simulink model "untitled1"  (R2024b)
settings: Solver=VariableStepAuto  StartTime=0.0  StopTime=10.0  RelTol=1e-3
undefined symbols (not defined in the file): control, controlParams, ControlSampleTime, CriticalTiltAngle, DiscIntNeverNeededParam, dspblkCoreblockFVToolHelper, flightState, FWControlParams, FWTrimSpeed, gcbh, ReferenceFilterDen, ReferenceFilterNum, tilt_max, tilt_trim, TiltScheduleRate, uavParam, w_trim, WindDownRate
libraries: slpidlib x31, simulink x9
(part 2 of 5)

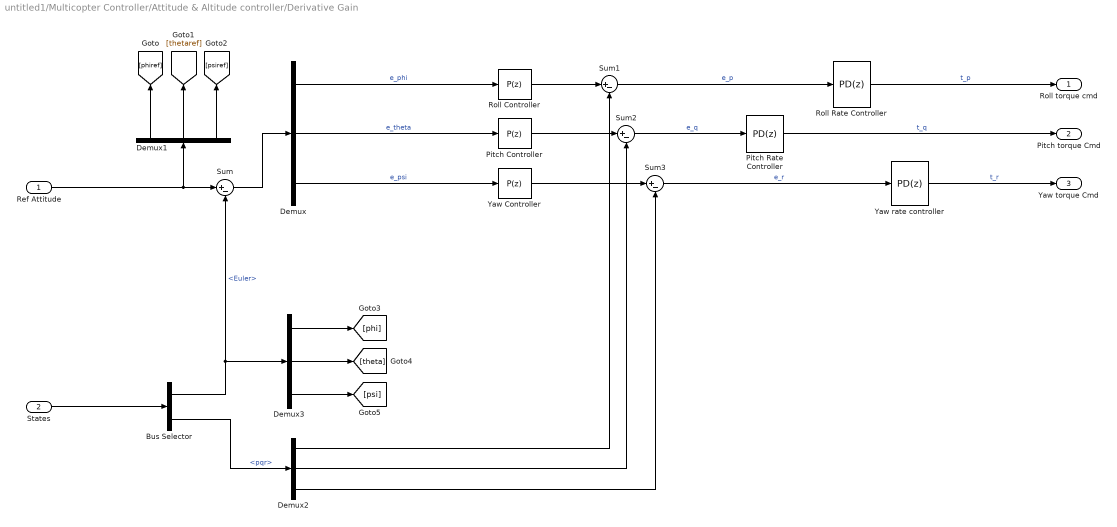
== system untitled1/Multicopter Controller/Attitude & Altitude controller/Derivative Gain ==
  Ref Attitude : Inport
  States : Inport  Port=2
  Bus Selector : BusSelector  OutputSignals=Euler,pqr
  Demux{,1..3} (4 alike) : Demux  Outputs=3
  Pitch Controller : slpidlib/PID Controller  Controller=P  Form=Parallel  TimeDomain=Discrete-time  UseExternalTs=off  SampleTime=0.005  IntegratorMethod=Forward Euler  FilterMethod=Forward Euler  ControllerParametersSource=internal  P=controlParams.P_PITCH  I=0.005  UseKiTs=on  D=1.47243904216696  UseExternalDerivativeSource=off  N=36.4796619058829  UseFilter=on  TunerSelectOption=Transfer Function Based (PID Tuner App)  InitialConditionSource=internal  InitialConditionForIntegrator=0  InitialConditionForFilter=0  DifferentiatorICPrevScaledInput=0  ExternalReset=none  TrackingMode=off  Kt=1  LimitOutput=off  SatLimitsSource=internal  UpperSaturationLimit=inf  LowerSaturationLimit=-inf  LinearizeAsGain=on  AntiWindupMode=none  Kb=1  LimitIntegrator=off  UpperIntegratorSaturationLimit=inf  LowerIntegratorSaturationLimit=-inf  POutMin=[]  POutMax=[]  IOutMin=[]  IOutMax=[]  DOutMin=[]  DOutMax=[]  NOutMin=[]  NOutMax=[]  SumOutMin=[]  SumOutMax=[]  SaturationOutMin=[]  SaturationOutMax=[]  PParamMin=[]  PParamMax=[]  IParamMin=[]  IParamMax=[]  DParamMin=[]  DParamMax=[]  NParamMin=[]  NParamMax=[]  KbParamMin=[]  KbParamMax=[]  KtParamMin=[]  KtParamMax=[]  KbOutMin=[]  KbOutMax=[]  KtOutMin=[]  KtOutMax=[]  IntegratorOutMin=[]  IntegratorOutMax=[]  FilterOutMin=[]  FilterOutMax=[]  SumI1OutMin=[]  SumI1OutMax=[]  SumI2OutMin=[]  SumI2OutMax=[]  SumI3OutMin=[]  SumI3OutMax=[]  SumI4OutMin=[]  SumI4OutMax=[]  SumDOutMin=[]  SumDOutMax=[]  DifferentiatorOutMin=[]  DifferentiatorOutMax=[]  FilterDiffOutCoefMin=[]  FilterDiffOutCoefMax=[]  ReciprocalOutMin=[]  ReciprocalOutMax=[]  SumDenOutMin=[]  SumDenOutMax=[]  SumNumOutMin=[]  SumNumOutMax=[]  DivideOutMin=[]  DivideOutMax=[]  UdiffTsProdOutMin=[]  UdiffTsProdOutMax=[]  NTsProdOutMin=[]  NTsProdOutMax=[]  UintegralTsProdOutMin=[]  UintegralTsProdOutMax=[]  UngainTsProdOutMin=[]  UngainTsProdOutMax=[]  ClampingZeroOutDataTypeStr=Inherit: Inherit via back propagation  ClampingZeroOutMin=[]  ClampingZeroOutMax=[]  FilterDenConstantOutDataTypeStr=Inherit: Inherit via back propagation  FilterDenConstantOutMin=[]  FilterDenConstantOutMax=[]  PCopyOutDataTypeStr=Inherit: Inherit via back propagation  PCopyOutMin=[]  PCopyOutMax=[]  NCopyOutDataTypeStr=Inherit: Inherit via back propagation  NCopyOutMin=[]  NCopyOutMax=[]  IntegratorContinuousStateAttributes=''  IntegratorStateMustResolveToSignalObject=off  IntegratorRTWStateStorageClass=Auto  FilterContinuousStateAttributes=''  FilterStateMustResolveToSignalObject=off  FilterRTWStateStorageClass=Auto  ParallelPVariant=InternalParameters  IdealPVariant=Disabled  IVariant=Disabled  DVariant=Disabled  IntegratorVariant=Disabled  SatVariant=Disabled  AWVariant=Disabled  PCopyVariant=Disabled  TRVariant=Disabled  FdbkBlocksVariant=Forward  IdealPFdbkVariant=Disabled  SatFdbkVariant=Disabled  DerivativeFilterVariant=Disabled  NVariant=Disabled  NCopyVariant=Disabled_SignalSpec  FilterICVariant=Disabled  IntegratorICVariant=Disabled  ExternalResetVariant=Disabled  TRSumVariant=Passthrough  SumFdbkVariant=Disabled  SumVariant=Passthrough_P  TsampFilterVariant=InternalTs  TsampNgainVariant=Passthrough  TsampIntegralVariant=Disabled_SignalSpec  ExternalSaturationOutDataTypeStr=Inherit: Same as second input  DerivativeSourceVariant=Disabled  PreIntVariant=InternalPreInt
  Pitch Rate Controller : slpidlib/PID Controller  Controller=PD  Form=Parallel  TimeDomain=Discrete-time  UseExternalTs=off  SampleTime=0.005  IntegratorMethod=Forward Euler  FilterMethod=Forward Euler  ControllerParametersSource=internal  P=controlParams.P_PITCH_RATE  I=controlParams.I_PITCH_RATE*0  UseKiTs=off  D=controlParams.D_PITCH_RATE  UseExternalDerivativeSource=off  N=controlParams.N_PITCH_RATE  UseFilter=on  TunerSelectOption=Transfer Function Based (PID Tuner App)  InitialConditionSource=internal  InitialConditionForIntegrator=0  InitialConditionForFilter=0  DifferentiatorICPrevScaledInput=0  ExternalReset=none  TrackingMode=off  Kt=1  LimitOutput=off  SatLimitsSource=internal  UpperSaturationLimit=inf  LowerSaturationLimit=-inf  LinearizeAsGain=on  AntiWindupMode=none  Kb=1  LimitIntegrator=off  UpperIntegratorSaturationLimit=inf  LowerIntegratorSaturationLimit=-inf  POutMin=[]  POutMax=[]  IOutMin=[]  IOutMax=[]  DOutMin=[]  DOutMax=[]  NOutMin=[]  NOutMax=[]  SumOutMin=[]  SumOutMax=[]  SaturationOutMin=[]  SaturationOutMax=[]  PParamMin=[]  PParamMax=[]  IParamMin=[]  IParamMax=[]  DParamMin=[]  DParamMax=[]  NParamMin=[]  NParamMax=[]  KbParamMin=[]  KbParamMax=[]  KtParamMin=[]  KtParamMax=[]  KbOutMin=[]  KbOutMax=[]  KtOutMin=[]  KtOutMax=[]  IntegratorOutMin=[]  IntegratorOutMax=[]  FilterOutMin=[]  FilterOutMax=[]  SumI1OutMin=[]  SumI1OutMax=[]  SumI2OutMin=[]  SumI2OutMax=[]  SumI3OutMin=[]  SumI3OutMax=[]  SumI4OutMin=[]  SumI4OutMax=[]  SumDOutMin=[]  SumDOutMax=[]  DifferentiatorOutMin=[]  DifferentiatorOutMax=[]  FilterDiffOutCoefMin=[]  FilterDiffOutCoefMax=[]  ReciprocalOutMin=[]  ReciprocalOutMax=[]  SumDenOutMin=[]  SumDenOutMax=[]  SumNumOutMin=[]  SumNumOutMax=[]  DivideOutMin=[]  DivideOutMax=[]  UdiffTsProdOutMin=[]  UdiffTsProdOutMax=[]  NTsProdOutMin=[]  NTsProdOutMax=[]  UintegralTsProdOutMin=[]  UintegralTsProdOutMax=[]  UngainTsProdOutMin=[]  UngainTsProdOutMax=[]  ClampingZeroOutDataTypeStr=Inherit: Inherit via back propagation  ClampingZeroOutMin=[]  ClampingZeroOutMax=[]  FilterDenConstantOutDataTypeStr=Inherit: Inherit via back propagation  FilterDenConstantOutMin=[]  FilterDenConstantOutMax=[]  PCopyOutDataTypeStr=Inherit: Inherit via back propagation  PCopyOutMin=[]  PCopyOutMax=[]  NCopyOutDataTypeStr=Inherit: Inherit via back propagation  NCopyOutMin=[]  NCopyOutMax=[]  IntegratorContinuousStateAttributes=''  IntegratorStateMustResolveToSignalObject=off  IntegratorRTWStateStorageClass=Auto  FilterContinuousStateAttributes=''  FilterStateMustResolveToSignalObject=off  FilterRTWStateStorageClass=Auto  ParallelPVariant=InternalParameters  IdealPVariant=Disabled  IVariant=Disabled  DVariant=InternalParameters  IntegratorVariant=Disabled  SatVariant=Disabled  AWVariant=Disabled  PCopyVariant=Disabled  TRVariant=Disabled  FdbkBlocksVariant=Forward  IdealPFdbkVariant=Disabled  SatFdbkVariant=Disabled  DerivativeFilterVariant=ForwardEulerFilter  NVariant=InternalParameters  NCopyVariant=Disabled  FilterICVariant=InternalICsFilter  IntegratorICVariant=Disabled  ExternalResetVariant=Disabled  TRSumVariant=Passthrough  SumFdbkVariant=Disabled  SumVariant=Sum_PD  TsampFilterVariant=InternalTs  TsampNgainVariant=Passthrough  TsampIntegralVariant=Disabled_SignalSpec  ExternalSaturationOutDataTypeStr=Inherit: Same as second input  DerivativeSourceVariant=ErrorSignal  PreIntVariant=InternalPreInt
  Roll Controller : slpidlib/PID Controller  Controller=P  Form=Parallel  TimeDomain=Discrete-time  UseExternalTs=off  SampleTime=0.005  IntegratorMethod=Forward Euler  FilterMethod=Forward Euler  ControllerParametersSource=internal  P=controlParams.P_ROLL  I=0.005  UseKiTs=on  D=0.952146167984845  UseExternalDerivativeSource=off  N=4.97655809990509  UseFilter=on  TunerSelectOption=Transfer Function Based (PID Tuner App)  InitialConditionSource=internal  InitialConditionForIntegrator=0  InitialConditionForFilter=0  DifferentiatorICPrevScaledInput=0  ExternalReset=none  TrackingMode=off  Kt=1  LimitOutput=off  SatLimitsSource=internal  UpperSaturationLimit=inf  LowerSaturationLimit=-inf  LinearizeAsGain=on  AntiWindupMode=none  Kb=1  LimitIntegrator=off  UpperIntegratorSaturationLimit=inf  LowerIntegratorSaturationLimit=-inf  POutMin=[]  POutMax=[]  IOutMin=[]  IOutMax=[]  DOutMin=[]  DOutMax=[]  NOutMin=[]  NOutMax=[]  SumOutMin=[]  SumOutMax=[]  SaturationOutMin=[]  SaturationOutMax=[]  PParamMin=[]  PParamMax=[]  IParamMin=[]  IParamMax=[]  DParamMin=[]  DParamMax=[]  NParamMin=[]  NParamMax=[]  KbParamMin=[]  KbParamMax=[]  KtParamMin=[]  KtParamMax=[]  KbOutMin=[]  KbOutMax=[]  KtOutMin=[]  KtOutMax=[]  IntegratorOutMin=[]  IntegratorOutMax=[]  FilterOutMin=[]  FilterOutMax=[]  SumI1OutMin=[]  SumI1OutMax=[]  SumI2OutMin=[]  SumI2OutMax=[]  SumI3OutMin=[]  SumI3OutMax=[]  SumI4OutMin=[]  SumI4OutMax=[]  SumDOutMin=[]  SumDOutMax=[]  DifferentiatorOutMin=[]  DifferentiatorOutMax=[]  FilterDiffOutCoefMin=[]  FilterDiffOutCoefMax=[]  ReciprocalOutMin=[]  ReciprocalOutMax=[]  SumDenOutMin=[]  SumDenOutMax=[]  SumNumOutMin=[]  SumNumOutMax=[]  DivideOutMin=[]  DivideOutMax=[]  UdiffTsProdOutMin=[]  UdiffTsProdOutMax=[]  NTsProdOutMin=[]  NTsProdOutMax=[]  UintegralTsProdOutMin=[]  UintegralTsProdOutMax=[]  UngainTsProdOutMin=[]  UngainTsProdOutMax=[]  ClampingZeroOutDataTypeStr=Inherit: Inherit via back propagation  ClampingZeroOutMin=[]  ClampingZeroOutMax=[]  FilterDenConstantOutDataTypeStr=Inherit: Inherit via back propagation  FilterDenConstantOutMin=[]  FilterDenConstantOutMax=[]  PCopyOutDataTypeStr=Inherit: Inherit via back propagation  PCopyOutMin=[]  PCopyOutMax=[]  NCopyOutDataTypeStr=Inherit: Inherit via back propagation  NCopyOutMin=[]  NCopyOutMax=[]  IntegratorContinuousStateAttributes=''  IntegratorStateMustResolveToSignalObject=off  IntegratorRTWStateStorageClass=Auto  FilterContinuousStateAttributes=''  FilterStateMustResolveToSignalObject=off  FilterRTWStateStorageClass=Auto  ParallelPVariant=InternalParameters  IdealPVariant=Disabled  IVariant=Disabled  DVariant=Disabled  IntegratorVariant=Disabled  SatVariant=Disabled  AWVariant=Disabled  PCopyVariant=Disabled  TRVariant=Disabled  FdbkBlocksVariant=Forward  IdealPFdbkVariant=Disabled  SatFdbkVariant=Disabled  DerivativeFilterVariant=Disabled  NVariant=Disabled  NCopyVariant=Disabled_SignalSpec  FilterICVariant=Disabled  IntegratorICVariant=Disabled  ExternalResetVariant=Disabled  TRSumVariant=Passthrough  SumFdbkVariant=Disabled  SumVariant=Passthrough_P  TsampFilterVariant=InternalTs  TsampNgainVariant=Passthrough  TsampIntegralVariant=Disabled_SignalSpec  ExternalSaturationOutDataTypeStr=Inherit: Same as second input  DerivativeSourceVariant=Disabled  PreIntVariant=InternalPreInt
  Roll Rate Controller : slpidlib/PID Controller  Controller=PD  Form=Parallel  TimeDomain=Discrete-time  UseExternalTs=off  SampleTime=-1  IntegratorMethod=Forward Euler  FilterMethod=Forward Euler  ControllerParametersSource=internal  P=controlParams.P_ROLL_RATE  I=controlParams.I_ROLL_RATE  UseKiTs=off  D=controlParams.D_ROLL_RATE  UseExternalDerivativeSource=off  N=controlParams.N_ROLL_RATE  UseFilter=on  TunerSelectOption=Transfer Function Based (PID Tuner App)  InitialConditionSource=internal  InitialConditionForIntegrator=0  InitialConditionForFilter=0  DifferentiatorICPrevScaledInput=0  ExternalReset=none  TrackingMode=off  Kt=1  LimitOutput=off  SatLimitsSource=internal  UpperSaturationLimit=inf  LowerSaturationLimit=-inf  LinearizeAsGain=on  AntiWindupMode=none  Kb=1  LimitIntegrator=off  UpperIntegratorSaturationLimit=inf  LowerIntegratorSaturationLimit=-inf  POutMin=[]  POutMax=[]  IOutMin=[]  IOutMax=[]  DOutMin=[]  DOutMax=[]  NOutMin=[]  NOutMax=[]  SumOutMin=[]  SumOutMax=[]  SaturationOutMin=[]  SaturationOutMax=[]  PParamMin=[]  PParamMax=[]  IParamMin=[]  IParamMax=[]  DParamMin=[]  DParamMax=[]  NParamMin=[]  NParamMax=[]  KbParamMin=[]  KbParamMax=[]  KtParamMin=[]  KtParamMax=[]  KbOutMin=[]  KbOutMax=[]  KtOutMin=[]  KtOutMax=[]  IntegratorOutMin=[]  IntegratorOutMax=[]  FilterOutMin=[]  FilterOutMax=[]  SumI1OutMin=[]  SumI1OutMax=[]  SumI2OutMin=[]  SumI2OutMax=[]  SumI3OutMin=[]  SumI3OutMax=[]  SumI4OutMin=[]  SumI4OutMax=[]  SumDOutMin=[]  SumDOutMax=[]  DifferentiatorOutMin=[]  DifferentiatorOutMax=[]  FilterDiffOutCoefMin=[]  FilterDiffOutCoefMax=[]  ReciprocalOutMin=[]  ReciprocalOutMax=[]  SumDenOutMin=[]  SumDenOutMax=[]  SumNumOutMin=[]  SumNumOutMax=[]  DivideOutMin=[]  DivideOutMax=[]  UdiffTsProdOutMin=[]  UdiffTsProdOutMax=[]  NTsProdOutMin=[]  NTsProdOutMax=[]  UintegralTsProdOutMin=[]  UintegralTsProdOutMax=[]  UngainTsProdOutMin=[]  UngainTsProdOutMax=[]  ClampingZeroOutDataTypeStr=Inherit: Inherit via back propagation  ClampingZeroOutMin=[]  ClampingZeroOutMax=[]  FilterDenConstantOutDataTypeStr=Inherit: Inherit via back propagation  FilterDenConstantOutMin=[]  FilterDenConstantOutMax=[]  PCopyOutDataTypeStr=Inherit: Inherit via back propagation  PCopyOutMin=[]  PCopyOutMax=[]  NCopyOutDataTypeStr=Inherit: Inherit via back propagation  NCopyOutMin=[]  NCopyOutMax=[]  IntegratorContinuousStateAttributes=''  IntegratorStateMustResolveToSignalObject=off  IntegratorRTWStateStorageClass=Auto  FilterContinuousStateAttributes=''  FilterStateMustResolveToSignalObject=off  FilterRTWStateStorageClass=Auto  ParallelPVariant=InternalParameters  IdealPVariant=Disabled  IVariant=Disabled  DVariant=InternalParameters  IntegratorVariant=Disabled  SatVariant=Disabled  AWVariant=Disabled  PCopyVariant=Disabled  TRVariant=Disabled  FdbkBlocksVariant=Forward  IdealPFdbkVariant=Disabled  SatFdbkVariant=Disabled  DerivativeFilterVariant=ForwardEulerFilter  NVariant=InternalParameters  NCopyVariant=Disabled  FilterICVariant=InternalICsFilter  IntegratorICVariant=Disabled  ExternalResetVariant=Disabled  TRSumVariant=Passthrough  SumFdbkVariant=Disabled  SumVariant=Sum_PD  TsampFilterVariant=InternalTs  TsampNgainVariant=Passthrough  TsampIntegralVariant=Disabled_SignalSpec  ExternalSaturationOutDataTypeStr=Inherit: Same as second input  DerivativeSourceVariant=ErrorSignal  PreIntVariant=InternalPreInt
  Sum{,1..3} (4 alike) : Sum  Inputs=|+-
  Yaw Controller : slpidlib/PID Controller  Controller=P  Form=Parallel  TimeDomain=Discrete-time  UseExternalTs=off  SampleTime=-1  IntegratorMethod=Forward Euler  FilterMethod=Forward Euler  ControllerParametersSource=internal  P=controlParams.P_YAW  I=0.005  UseKiTs=off  D=1.48888612768425  UseExternalDerivativeSource=off  N=213.334111142952  UseFilter=on  TunerSelectOption=Transfer Function Based (PID Tuner App)  InitialConditionSource=internal  InitialConditionForIntegrator=0  InitialConditionForFilter=0  DifferentiatorICPrevScaledInput=0  ExternalReset=none  TrackingMode=off  Kt=1  LimitOutput=off  SatLimitsSource=internal  UpperSaturationLimit=inf  LowerSaturationLimit=-inf  LinearizeAsGain=on  AntiWindupMode=none  Kb=1  LimitIntegrator=off  UpperIntegratorSaturationLimit=inf  LowerIntegratorSaturationLimit=-inf  POutMin=[]  POutMax=[]  IOutMin=[]  IOutMax=[]  DOutMin=[]  DOutMax=[]  NOutMin=[]  NOutMax=[]  SumOutMin=[]  SumOutMax=[]  SaturationOutMin=[]  SaturationOutMax=[]  PParamMin=[]  PParamMax=[]  IParamMin=[]  IParamMax=[]  DParamMin=[]  DParamMax=[]  NParamMin=[]  NParamMax=[]  KbParamMin=[]  KbParamMax=[]  KtParamMin=[]  KtParamMax=[]  KbOutMin=[]  KbOutMax=[]  KtOutMin=[]  KtOutMax=[]  IntegratorOutMin=[]  IntegratorOutMax=[]  FilterOutMin=[]  FilterOutMax=[]  SumI1OutMin=[]  SumI1OutMax=[]  SumI2OutMin=[]  SumI2OutMax=[]  SumI3OutMin=[]  SumI3OutMax=[]  SumI4OutMin=[]  SumI4OutMax=[]  SumDOutMin=[]  SumDOutMax=[]  DifferentiatorOutMin=[]  DifferentiatorOutMax=[]  FilterDiffOutCoefMin=[]  FilterDiffOutCoefMax=[]  ReciprocalOutMin=[]  ReciprocalOutMax=[]  SumDenOutMin=[]  SumDenOutMax=[]  SumNumOutMin=[]  SumNumOutMax=[]  DivideOutMin=[]  DivideOutMax=[]  UdiffTsProdOutMin=[]  UdiffTsProdOutMax=[]  NTsProdOutMin=[]  NTsProdOutMax=[]  UintegralTsProdOutMin=[]  UintegralTsProdOutMax=[]  UngainTsProdOutMin=[]  UngainTsProdOutMax=[]  ClampingZeroOutDataTypeStr=Inherit: Inherit via back propagation  ClampingZeroOutMin=[]  ClampingZeroOutMax=[]  FilterDenConstantOutDataTypeStr=Inherit: Inherit via back propagation  FilterDenConstantOutMin=[]  FilterDenConstantOutMax=[]  PCopyOutDataTypeStr=Inherit: Inherit via back propagation  PCopyOutMin=[]  PCopyOutMax=[]  NCopyOutDataTypeStr=Inherit: Inherit via back propagation  NCopyOutMin=[]  NCopyOutMax=[]  IntegratorContinuousStateAttributes=''  IntegratorStateMustResolveToSignalObject=off  IntegratorRTWStateStorageClass=Auto  FilterContinuousStateAttributes=''  FilterStateMustResolveToSignalObject=off  FilterRTWStateStorageClass=Auto  ParallelPVariant=InternalParameters  IdealPVariant=Disabled  IVariant=Disabled  DVariant=Disabled  IntegratorVariant=Disabled  SatVariant=Disabled  AWVariant=Disabled  PCopyVariant=Disabled  TRVariant=Disabled  FdbkBlocksVariant=Forward  IdealPFdbkVariant=Disabled  SatFdbkVariant=Disabled  DerivativeFilterVariant=Disabled  NVariant=Disabled  NCopyVariant=Disabled_SignalSpec  FilterICVariant=Disabled  IntegratorICVariant=Disabled  ExternalResetVariant=Disabled  TRSumVariant=Passthrough  SumFdbkVariant=Disabled  SumVariant=Passthrough_P  TsampFilterVariant=InternalTs  TsampNgainVariant=Passthrough  TsampIntegralVariant=Disabled_SignalSpec  ExternalSaturationOutDataTypeStr=Inherit: Same as second input  DerivativeSourceVariant=Disabled  PreIntVariant=InternalPreInt
  Yaw rate controller : slpidlib/PID Controller  Controller=PD  Form=Parallel  TimeDomain=Discrete-time  UseExternalTs=off  SampleTime=-1  IntegratorMethod=Forward Euler  FilterMethod=Forward Euler  ControllerParametersSource=internal  P=controlParams.P_YAW_RATE  I=controlParams.I_YAW_RATE  UseKiTs=off  D=controlParams.D_YAW_RATE  UseExternalDerivativeSource=off  N=controlParams.N_YAW_RATE  UseFilter=on  TunerSelectOption=Transfer Function Based (PID Tuner App)  InitialConditionSource=internal  InitialConditionForIntegrator=0  InitialConditionForFilter=0  DifferentiatorICPrevScaledInput=0  ExternalReset=none  TrackingMode=off  Kt=1  LimitOutput=off  SatLimitsSource=internal  UpperSaturationLimit=inf  LowerSaturationLimit=-inf  LinearizeAsGain=on  AntiWindupMode=none  Kb=1  LimitIntegrator=off  UpperIntegratorSaturationLimit=inf  LowerIntegratorSaturationLimit=-inf  POutMin=[]  POutMax=[]  IOutMin=[]  IOutMax=[]  DOutMin=[]  DOutMax=[]  NOutMin=[]  NOutMax=[]  SumOutMin=[]  SumOutMax=[]  SaturationOutMin=[]  SaturationOutMax=[]  PParamMin=[]  PParamMax=[]  IParamMin=[]  IParamMax=[]  DParamMin=[]  DParamMax=[]  NParamMin=[]  NParamMax=[]  KbParamMin=[]  KbParamMax=[]  KtParamMin=[]  KtParamMax=[]  KbOutMin=[]  KbOutMax=[]  KtOutMin=[]  KtOutMax=[]  IntegratorOutMin=[]  IntegratorOutMax=[]  FilterOutMin=[]  FilterOutMax=[]  SumI1OutMin=[]  SumI1OutMax=[]  SumI2OutMin=[]  SumI2OutMax=[]  SumI3OutMin=[]  SumI3OutMax=[]  SumI4OutMin=[]  SumI4OutMax=[]  SumDOutMin=[]  SumDOutMax=[]  DifferentiatorOutMin=[]  DifferentiatorOutMax=[]  FilterDiffOutCoefMin=[]  FilterDiffOutCoefMax=[]  ReciprocalOutMin=[]  ReciprocalOutMax=[]  SumDenOutMin=[]  SumDenOutMax=[]  SumNumOutMin=[]  SumNumOutMax=[]  DivideOutMin=[]  DivideOutMax=[]  UdiffTsProdOutMin=[]  UdiffTsProdOutMax=[]  NTsProdOutMin=[]  NTsProdOutMax=[]  UintegralTsProdOutMin=[]  UintegralTsProdOutMax=[]  UngainTsProdOutMin=[]  UngainTsProdOutMax=[]  ClampingZeroOutDataTypeStr=Inherit: Inherit via back propagation  ClampingZeroOutMin=[]  ClampingZeroOutMax=[]  FilterDenConstantOutDataTypeStr=Inherit: Inherit via back propagation  FilterDenConstantOutMin=[]  FilterDenConstantOutMax=[]  PCopyOutDataTypeStr=Inherit: Inherit via back propagation  PCopyOutMin=[]  PCopyOutMax=[]  NCopyOutDataTypeStr=Inherit: Inherit via back propagation  NCopyOutMin=[]  NCopyOutMax=[]  IntegratorContinuousStateAttributes=''  IntegratorStateMustResolveToSignalObject=off  IntegratorRTWStateStorageClass=Auto  FilterContinuousStateAttributes=''  FilterStateMustResolveToSignalObject=off  FilterRTWStateStorageClass=Auto  ParallelPVariant=InternalParameters  IdealPVariant=Disabled  IVariant=Disabled  DVariant=InternalParameters  IntegratorVariant=Disabled  SatVariant=Disabled  AWVariant=Disabled  PCopyVariant=Disabled  TRVariant=Disabled  FdbkBlocksVariant=Forward  IdealPFdbkVariant=Disabled  SatFdbkVariant=Disabled  DerivativeFilterVariant=ForwardEulerFilter  NVariant=InternalParameters  NCopyVariant=Disabled  FilterICVariant=InternalICsFilter  IntegratorICVariant=Disabled  ExternalResetVariant=Disabled  TRSumVariant=Passthrough  SumFdbkVariant=Disabled  SumVariant=Sum_PD  TsampFilterVariant=InternalTs  TsampNgainVariant=Passthrough  TsampIntegralVariant=Disabled_SignalSpec  ExternalSaturationOutDataTypeStr=Inherit: Same as second input  DerivativeSourceVariant=ErrorSignal  PreIntVariant=InternalPreInt
  Roll torque cmd : Outport
  Pitch torque Cmd : Outport  Port=2
  Yaw torque Cmd : Outport  Port=3
  wires:
  Sum/1 -> Demux/1
  Demux/1 -> Roll Controller/1  "e_phi"
  Sum1/1 -> Roll Rate Controller/1  "e_p"
  Demux1/1 -> [phiref]
  Demux1/2 -> [thetaref]
  Demux1/3 -> [psiref]
  Bus Selector/1 -> Demux3/1, Sum/2  "<Euler>"
  Demux2/2 -> Sum2/2
  Demux3/1 -> [phi]
  Demux3/2 -> [theta]
  Demux3/3 -> [psi]
  Bus Selector/2 -> Demux2/1  "<pqr>"
  Sum2/1 -> Pitch Rate Controller/1  "e_q"
  Demux2/3 -> Sum3/2
  Demux2/1 -> Sum1/2
  Roll Controller/1 -> Sum1/1
  States/1 -> Bus Selector/1
  Ref Attitude/1 -> Demux1/1, Sum/1
  Roll Rate Controller/1 -> Roll torque cmd/1  "t_p"
  Pitch Rate Controller/1 -> Pitch torque Cmd/1  "t_q"
  Demux/2 -> Pitch Controller/1  "e_theta"
  Pitch Controller/1 -> Sum2/1
  Demux/3 -> Yaw Controller/1  "e_psi"
  Yaw Controller/1 -> Sum3/1
  Sum3/1 -> Yaw rate controller/1  "e_r"
  Yaw rate controller/1 -> Yaw torque Cmd/1  "t_r"

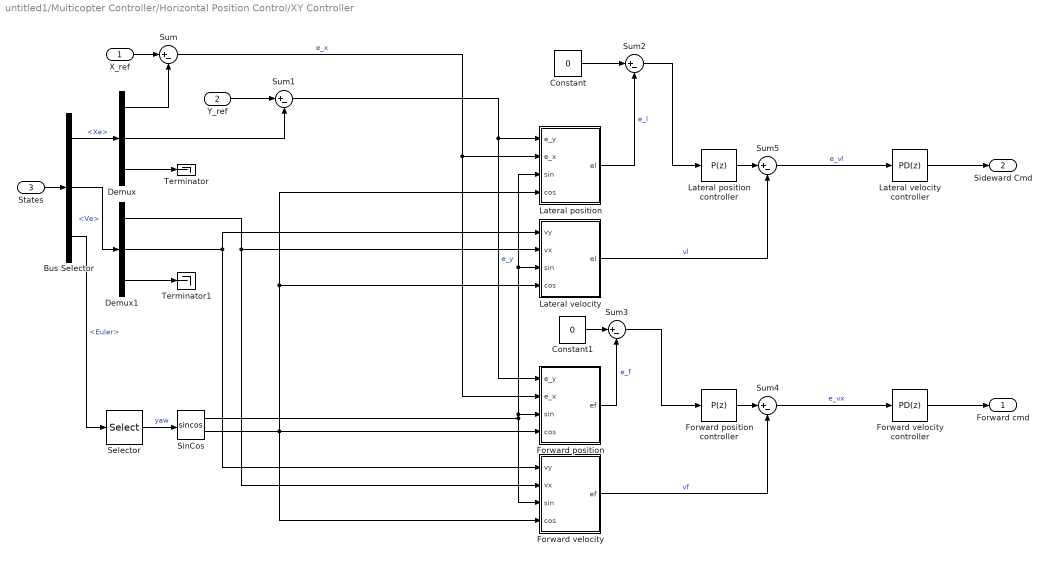
== system untitled1/Multicopter Controller/Horizontal Position Control/XY Controller ==
  X_ref : Inport
  Y_ref : Inport  Port=2
  States : Inport  Port=3
  Bus Selector : BusSelector  OutputSignals=Xe,Ve,Euler
  Constant : Constant  Value=0
  Constant1 : Constant  Value=0
  Demux : Demux  Outputs=3
  Demux1 : Demux  Outputs=3
  Forward position : Subsystem
  Forward position controller : slpidlib/PID Controller  Controller=P  Form=Parallel  TimeDomain=Discrete-time  UseExternalTs=off  SampleTime=-1  IntegratorMethod=Forward Euler  FilterMethod=Forward Euler  ControllerParametersSource=internal  P=controlParams.P_X  I=controlParams.I_X  UseKiTs=off  D=0.741088334151374  UseExternalDerivativeSource=off  N=1.14081860742283  UseFilter=on  TunerSelectOption=Transfer Function Based (PID Tuner App)  InitialConditionSource=internal  InitialConditionForIntegrator=0  InitialConditionForFilter=0  DifferentiatorICPrevScaledInput=0  ExternalReset=none  TrackingMode=off  Kt=1  LimitOutput=off  SatLimitsSource=internal  UpperSaturationLimit=inf  LowerSaturationLimit=-inf  LinearizeAsGain=on  AntiWindupMode=none  Kb=1  LimitIntegrator=off  UpperIntegratorSaturationLimit=inf  LowerIntegratorSaturationLimit=-inf  POutMin=[]  POutMax=[]  IOutMin=[]  IOutMax=[]  DOutMin=[]  DOutMax=[]  NOutMin=[]  NOutMax=[]  SumOutMin=[]  SumOutMax=[]  SaturationOutMin=[]  SaturationOutMax=[]  PParamMin=[]  PParamMax=[]  IParamMin=[]  IParamMax=[]  DParamMin=[]  DParamMax=[]  NParamMin=[]  NParamMax=[]  KbParamMin=[]  KbParamMax=[]  KtParamMin=[]  KtParamMax=[]  KbOutMin=[]  KbOutMax=[]  KtOutMin=[]  KtOutMax=[]  IntegratorOutMin=[]  IntegratorOutMax=[]  FilterOutMin=[]  FilterOutMax=[]  SumI1OutMin=[]  SumI1OutMax=[]  SumI2OutMin=[]  SumI2OutMax=[]  SumI3OutMin=[]  SumI3OutMax=[]  SumI4OutMin=[]  SumI4OutMax=[]  SumDOutMin=[]  SumDOutMax=[]  DifferentiatorOutMin=[]  DifferentiatorOutMax=[]  FilterDiffOutCoefMin=[]  FilterDiffOutCoefMax=[]  ReciprocalOutMin=[]  ReciprocalOutMax=[]  SumDenOutMin=[]  SumDenOutMax=[]  SumNumOutMin=[]  SumNumOutMax=[]  DivideOutMin=[]  DivideOutMax=[]  UdiffTsProdOutMin=[]  UdiffTsProdOutMax=[]  NTsProdOutMin=[]  NTsProdOutMax=[]  UintegralTsProdOutMin=[]  UintegralTsProdOutMax=[]  UngainTsProdOutMin=[]  UngainTsProdOutMax=[]  ClampingZeroOutDataTypeStr=Inherit: Inherit via back propagation  ClampingZeroOutMin=[]  ClampingZeroOutMax=[]  FilterDenConstantOutDataTypeStr=Inherit: Inherit via back propagation  FilterDenConstantOutMin=[]  FilterDenConstantOutMax=[]  PCopyOutDataTypeStr=Inherit: Inherit via back propagation  PCopyOutMin=[]  PCopyOutMax=[]  NCopyOutDataTypeStr=Inherit: Inherit via back propagation  NCopyOutMin=[]  NCopyOutMax=[]  IntegratorContinuousStateAttributes=''  IntegratorStateMustResolveToSignalObject=off  IntegratorRTWStateStorageClass=Auto  FilterContinuousStateAttributes=''  FilterStateMustResolveToSignalObject=off  FilterRTWStateStorageClass=Auto  ParallelPVariant=InternalParameters  IdealPVariant=Disabled  IVariant=Disabled  DVariant=Disabled  IntegratorVariant=Disabled  SatVariant=Disabled  AWVariant=Disabled  PCopyVariant=Disabled  TRVariant=Disabled  FdbkBlocksVariant=Forward  IdealPFdbkVariant=Disabled  SatFdbkVariant=Disabled  DerivativeFilterVariant=Disabled  NVariant=Disabled  NCopyVariant=Disabled_SignalSpec  FilterICVariant=Disabled  IntegratorICVariant=Disabled  ExternalResetVariant=Disabled  TRSumVariant=Passthrough  SumFdbkVariant=Disabled  SumVariant=Passthrough_P  TsampFilterVariant=InternalTs  TsampNgainVariant=Passthrough  TsampIntegralVariant=Disabled_SignalSpec  ExternalSaturationOutDataTypeStr=Inherit: Same as second input  DerivativeSourceVariant=Disabled  PreIntVariant=InternalPreInt
  Forward velocity : Subsystem
  Forward velocity controller : slpidlib/PID Controller  Controller=PD  Form=Parallel  TimeDomain=Discrete-time  UseExternalTs=off  SampleTime=-1  IntegratorMethod=Forward Euler  FilterMethod=Forward Euler  ControllerParametersSource=internal  P=controlParams.P_VX  I=0  UseKiTs=off  D=controlParams.D_VX  UseExternalDerivativeSource=off  N=controlParams.N_VX  UseFilter=on  TunerSelectOption=Transfer Function Based (PID Tuner App)  InitialConditionSource=internal  InitialConditionForIntegrator=0  InitialConditionForFilter=0  DifferentiatorICPrevScaledInput=0  ExternalReset=none  TrackingMode=off  Kt=1  LimitOutput=off  SatLimitsSource=internal  UpperSaturationLimit=inf  LowerSaturationLimit=-inf  LinearizeAsGain=on  AntiWindupMode=none  Kb=1  LimitIntegrator=off  UpperIntegratorSaturationLimit=inf  LowerIntegratorSaturationLimit=-inf  POutMin=[]  POutMax=[]  IOutMin=[]  IOutMax=[]  DOutMin=[]  DOutMax=[]  NOutMin=[]  NOutMax=[]  SumOutMin=[]  SumOutMax=[]  SaturationOutMin=[]  SaturationOutMax=[]  PParamMin=[]  PParamMax=[]  IParamMin=[]  IParamMax=[]  DParamMin=[]  DParamMax=[]  NParamMin=[]  NParamMax=[]  KbParamMin=[]  KbParamMax=[]  KtParamMin=[]  KtParamMax=[]  KbOutMin=[]  KbOutMax=[]  KtOutMin=[]  KtOutMax=[]  IntegratorOutMin=[]  IntegratorOutMax=[]  FilterOutMin=[]  FilterOutMax=[]  SumI1OutMin=[]  SumI1OutMax=[]  SumI2OutMin=[]  SumI2OutMax=[]  SumI3OutMin=[]  SumI3OutMax=[]  SumI4OutMin=[]  SumI4OutMax=[]  SumDOutMin=[]  SumDOutMax=[]  DifferentiatorOutMin=[]  DifferentiatorOutMax=[]  FilterDiffOutCoefMin=[]  FilterDiffOutCoefMax=[]  ReciprocalOutMin=[]  ReciprocalOutMax=[]  SumDenOutMin=[]  SumDenOutMax=[]  SumNumOutMin=[]  SumNumOutMax=[]  DivideOutMin=[]  DivideOutMax=[]  UdiffTsProdOutMin=[]  UdiffTsProdOutMax=[]  NTsProdOutMin=[]  NTsProdOutMax=[]  UintegralTsProdOutMin=[]  UintegralTsProdOutMax=[]  UngainTsProdOutMin=[]  UngainTsProdOutMax=[]  ClampingZeroOutDataTypeStr=Inherit: Inherit via back propagation  ClampingZeroOutMin=[]  ClampingZeroOutMax=[]  FilterDenConstantOutDataTypeStr=Inherit: Inherit via back propagation  FilterDenConstantOutMin=[]  FilterDenConstantOutMax=[]  PCopyOutDataTypeStr=Inherit: Inherit via back propagation  PCopyOutMin=[]  PCopyOutMax=[]  NCopyOutDataTypeStr=Inherit: Inherit via back propagation  NCopyOutMin=[]  NCopyOutMax=[]  IntegratorContinuousStateAttributes=''  IntegratorStateMustResolveToSignalObject=off  IntegratorRTWStateStorageClass=Auto  FilterContinuousStateAttributes=''  FilterStateMustResolveToSignalObject=off  FilterRTWStateStorageClass=Auto  ParallelPVariant=InternalParameters  IdealPVariant=Disabled  IVariant=Disabled  DVariant=InternalParameters  IntegratorVariant=Disabled  SatVariant=Disabled  AWVariant=Disabled  PCopyVariant=Disabled  TRVariant=Disabled  FdbkBlocksVariant=Forward  IdealPFdbkVariant=Disabled  SatFdbkVariant=Disabled  DerivativeFilterVariant=ForwardEulerFilter  NVariant=InternalParameters  NCopyVariant=Disabled  FilterICVariant=InternalICsFilter  IntegratorICVariant=Disabled  ExternalResetVariant=Disabled  TRSumVariant=Passthrough  SumFdbkVariant=Disabled  SumVariant=Sum_PD  TsampFilterVariant=InternalTs  TsampNgainVariant=Passthrough  TsampIntegralVariant=Disabled_SignalSpec  ExternalSaturationOutDataTypeStr=Inherit: Same as second input  DerivativeSourceVariant=ErrorSignal  PreIntVariant=InternalPreInt
  Lateral position : Subsystem
  Lateral position controller : slpidlib/PID Controller  Controller=P  Form=Parallel  TimeDomain=Discrete-time  UseExternalTs=off  SampleTime=-1  IntegratorMethod=Forward Euler  FilterMethod=Forward Euler  ControllerParametersSource=internal  P=controlParams.P_Y  I=controlParams.I_Y  UseKiTs=off  D=0.20966837124708  UseExternalDerivativeSource=off  N=1.18305565097938  UseFilter=on  TunerSelectOption=Transfer Function Based (PID Tuner App)  InitialConditionSource=internal  InitialConditionForIntegrator=0  InitialConditionForFilter=0  DifferentiatorICPrevScaledInput=0  ExternalReset=none  TrackingMode=off  Kt=1  LimitOutput=off  SatLimitsSource=internal  UpperSaturationLimit=0.4  LowerSaturationLimit=-0.4  LinearizeAsGain=on  AntiWindupMode=clamping  Kb=1  LimitIntegrator=off  UpperIntegratorSaturationLimit=inf  LowerIntegratorSaturationLimit=-inf  POutMin=[]  POutMax=[]  IOutMin=[]  IOutMax=[]  DOutMin=[]  DOutMax=[]  NOutMin=[]  NOutMax=[]  SumOutMin=[]  SumOutMax=[]  SaturationOutMin=[]  SaturationOutMax=[]  PParamMin=[]  PParamMax=[]  IParamMin=[]  IParamMax=[]  DParamMin=[]  DParamMax=[]  NParamMin=[]  NParamMax=[]  KbParamMin=[]  KbParamMax=[]  KtParamMin=[]  KtParamMax=[]  KbOutMin=[]  KbOutMax=[]  KtOutMin=[]  KtOutMax=[]  IntegratorOutMin=[]  IntegratorOutMax=[]  FilterOutMin=[]  FilterOutMax=[]  SumI1OutMin=[]  SumI1OutMax=[]  SumI2OutMin=[]  SumI2OutMax=[]  SumI3OutMin=[]  SumI3OutMax=[]  SumI4OutMin=[]  SumI4OutMax=[]  SumDOutMin=[]  SumDOutMax=[]  DifferentiatorOutMin=[]  DifferentiatorOutMax=[]  FilterDiffOutCoefMin=[]  FilterDiffOutCoefMax=[]  ReciprocalOutMin=[]  ReciprocalOutMax=[]  SumDenOutMin=[]  SumDenOutMax=[]  SumNumOutMin=[]  SumNumOutMax=[]  DivideOutMin=[]  DivideOutMax=[]  UdiffTsProdOutMin=[]  UdiffTsProdOutMax=[]  NTsProdOutMin=[]  NTsProdOutMax=[]  UintegralTsProdOutMin=[]  UintegralTsProdOutMax=[]  UngainTsProdOutMin=[]  UngainTsProdOutMax=[]  ClampingZeroOutDataTypeStr=Inherit: Inherit via back propagation  ClampingZeroOutMin=[]  ClampingZeroOutMax=[]  FilterDenConstantOutDataTypeStr=Inherit: Inherit via back propagation  FilterDenConstantOutMin=[]  FilterDenConstantOutMax=[]  PCopyOutDataTypeStr=Inherit: Inherit via back propagation  PCopyOutMin=[]  PCopyOutMax=[]  NCopyOutDataTypeStr=Inherit: Inherit via back propagation  NCopyOutMin=[]  NCopyOutMax=[]  IntegratorContinuousStateAttributes=''  IntegratorStateMustResolveToSignalObject=off  IntegratorRTWStateStorageClass=Auto  FilterContinuousStateAttributes=''  FilterStateMustResolveToSignalObject=off  FilterRTWStateStorageClass=Auto  ParallelPVariant=InternalParameters  IdealPVariant=Disabled  IVariant=Disabled  DVariant=Disabled  IntegratorVariant=Disabled  SatVariant=Disabled  AWVariant=Disabled  PCopyVariant=Disabled  TRVariant=Disabled  FdbkBlocksVariant=Forward  IdealPFdbkVariant=Disabled  SatFdbkVariant=Disabled  DerivativeFilterVariant=Disabled  NVariant=Disabled  NCopyVariant=Disabled_SignalSpec  FilterICVariant=Disabled  IntegratorICVariant=Disabled  ExternalResetVariant=Disabled  TRSumVariant=Passthrough  SumFdbkVariant=Disabled  SumVariant=Passthrough_P  TsampFilterVariant=InternalTs  TsampNgainVariant=Passthrough  TsampIntegralVariant=Disabled_SignalSpec  ExternalSaturationOutDataTypeStr=Inherit: Same as second input  DerivativeSourceVariant=Disabled  PreIntVariant=InternalPreInt
  Lateral velocity : Subsystem
  "Lateral velocity controller " : slpidlib/PID Controller  Controller=PD  Form=Parallel  TimeDomain=Discrete-time  UseExternalTs=off  SampleTime=-1  IntegratorMethod=Forward Euler  FilterMethod=Forward Euler  ControllerParametersSource=internal  P=controlParams.P_VY  I=0  UseKiTs=off  D=controlParams.D_VY  UseExternalDerivativeSource=off  N=controlParams.N_VY  UseFilter=on  TunerSelectOption=Transfer Function Based (PID Tuner App)  InitialConditionSource=internal  InitialConditionForIntegrator=0  InitialConditionForFilter=0  DifferentiatorICPrevScaledInput=0  ExternalReset=none  TrackingMode=off  Kt=1  LimitOutput=off  SatLimitsSource=internal  UpperSaturationLimit=inf  LowerSaturationLimit=-inf  LinearizeAsGain=on  AntiWindupMode=none  Kb=1  LimitIntegrator=off  UpperIntegratorSaturationLimit=inf  LowerIntegratorSaturationLimit=-inf  POutMin=[]  POutMax=[]  IOutMin=[]  IOutMax=[]  DOutMin=[]  DOutMax=[]  NOutMin=[]  NOutMax=[]  SumOutMin=[]  SumOutMax=[]  SaturationOutMin=[]  SaturationOutMax=[]  PParamMin=[]  PParamMax=[]  IParamMin=[]  IParamMax=[]  DParamMin=[]  DParamMax=[]  NParamMin=[]  NParamMax=[]  KbParamMin=[]  KbParamMax=[]  KtParamMin=[]  KtParamMax=[]  KbOutMin=[]  KbOutMax=[]  KtOutMin=[]  KtOutMax=[]  IntegratorOutMin=[]  IntegratorOutMax=[]  FilterOutMin=[]  FilterOutMax=[]  SumI1OutMin=[]  SumI1OutMax=[]  SumI2OutMin=[]  SumI2OutMax=[]  SumI3OutMin=[]  SumI3OutMax=[]  SumI4OutMin=[]  SumI4OutMax=[]  SumDOutMin=[]  SumDOutMax=[]  DifferentiatorOutMin=[]  DifferentiatorOutMax=[]  FilterDiffOutCoefMin=[]  FilterDiffOutCoefMax=[]  ReciprocalOutMin=[]  ReciprocalOutMax=[]  SumDenOutMin=[]  SumDenOutMax=[]  SumNumOutMin=[]  SumNumOutMax=[]  DivideOutMin=[]  DivideOutMax=[]  UdiffTsProdOutMin=[]  UdiffTsProdOutMax=[]  NTsProdOutMin=[]  NTsProdOutMax=[]  UintegralTsProdOutMin=[]  UintegralTsProdOutMax=[]  UngainTsProdOutMin=[]  UngainTsProdOutMax=[]  ClampingZeroOutDataTypeStr=Inherit: Inherit via back propagation  ClampingZeroOutMin=[]  ClampingZeroOutMax=[]  FilterDenConstantOutDataTypeStr=Inherit: Inherit via back propagation  FilterDenConstantOutMin=[]  FilterDenConstantOutMax=[]  PCopyOutDataTypeStr=Inherit: Inherit via back propagation  PCopyOutMin=[]  PCopyOutMax=[]  NCopyOutDataTypeStr=Inherit: Inherit via back propagation  NCopyOutMin=[]  NCopyOutMax=[]  IntegratorContinuousStateAttributes=''  IntegratorStateMustResolveToSignalObject=off  IntegratorRTWStateStorageClass=Auto  FilterContinuousStateAttributes=''  FilterStateMustResolveToSignalObject=off  FilterRTWStateStorageClass=Auto  ParallelPVariant=InternalParameters  IdealPVariant=Disabled  IVariant=Disabled  DVariant=InternalParameters  IntegratorVariant=Disabled  SatVariant=Disabled  AWVariant=Disabled  PCopyVariant=Disabled  TRVariant=Disabled  FdbkBlocksVariant=Forward  IdealPFdbkVariant=Disabled  SatFdbkVariant=Disabled  DerivativeFilterVariant=ForwardEulerFilter  NVariant=InternalParameters  NCopyVariant=Disabled  FilterICVariant=InternalICsFilter  IntegratorICVariant=Disabled  ExternalResetVariant=Disabled  TRSumVariant=Passthrough  SumFdbkVariant=Disabled  SumVariant=Sum_PD  TsampFilterVariant=InternalTs  TsampNgainVariant=Passthrough  TsampIntegralVariant=Disabled_SignalSpec  ExternalSaturationOutDataTypeStr=Inherit: Same as second input  DerivativeSourceVariant=ErrorSignal  PreIntVariant=InternalPreInt
  Selector : Selector  InputPortWidth=3  IndexOptions=Index vector (dialog)  Indices=[3]  OutputSizes=1
  SinCos : Trigonometry  Operator=sincos
  Sum{,1..5} (6 alike) : Sum  Inputs=|+-
  Terminator : Terminator
  Terminator1 : Terminator
  Forward cmd : Outport
  Sideward Cmd : Outport  Port=2
  wires:
  Demux/1 -> Sum/2
  States/1 -> Bus Selector/1
  Bus Selector/1 -> Demux/1  "<Xe>"
  X_ref/1 -> Sum/1
  Bus Selector/2 -> Demux1/1  "<Ve>"
  Y_ref/1 -> Sum1/1
  Demux/2 -> Sum1/2
  Demux/3 -> Terminator/1
  Sum4/1 -> Forward velocity controller/1  "e_vx"
  SinCos/2 -> Forward velocity/4(cos), Lateral position/4(cos), Lateral velocity/4(cos), Forward position/4(cos)
  Selector/1 -> SinCos/1  "yaw"
  Lateral position/1(el) -> Sum2/2  "e_l"
  Sum1/1 -> Forward position/1(e_y), Lateral position/1(e_y)  "e_y"
  Sum/1 -> Forward position/2(e_x), Lateral position/2(e_x)  "e_x"
  Demux1/1 -> Forward velocity/2(vx), Lateral velocity/2(vx)
  Demux1/2 -> Forward velocity/1(vy), Lateral velocity/1(vy)
  Demux1/3 -> Terminator1/1
  SinCos/1 -> Lateral velocity/3(sin), Lateral position/3(sin), Forward position/3(sin), Forward velocity/3(sin)
  Lateral velocity/1(el) -> Sum5/2  "vl"
  Forward position/1(ef) -> Sum3/2  "e_f"
  Forward velocity/1(ef) -> Sum4/2  "vf"
  Lateral position controller/1 -> Sum5/1
  Forward position controller/1 -> Sum4/1
  Sum5/1 -> "Lateral velocity controller "/1  "e_vl"
  Bus Selector/3 -> Selector/1  "<Euler>"
  "Lateral velocity controller "/1 -> Sideward Cmd/1
  Forward velocity controller/1 -> Forward cmd/1
  Constant/1 -> Sum2/1
  Sum2/1 -> Lateral position controller/1
  Constant1/1 -> Sum3/1
  Sum3/1 -> Forward position controller/1

== system untitled1/Multicopter Controller/Subsystem/Triggered Subsystem ==
  YawHold : Inport
  Trigger : TriggerPort  VariantControl=(inherit)
  Reference : Outport
  wires:
  YawHold/1 -> Reference/1

== system untitled1/Scheduler/FixedWingScheduler/Switch Case Action Subsystem ==
  note: No control allocated from fixed wing during hover.
  Action Port : ActionPort
  Bus Creator : BusCreator  Inputs=4
  Constant{,1..3} (4 alike) : Constant  Value=0
  FixedWingControls : Outport  OutDataTypeStr=Bus: FixedWingCtrlBus
  wires:
  Bus Creator/1 -> FixedWingControls/1
  Constant/1 -> Bus Creator/1  "dA"
  Constant1/1 -> Bus Creator/2  "dE"
  Constant2/1 -> Bus Creator/3  "dR"
  Constant3/1 -> Bus Creator/4  "dT"

== system untitled1/Scheduler/FixedWingScheduler/Switch Case Action Subsystem1 ==
  FixedWingActuators : Inport  OutDataTypeStr=Bus: FixedWingCtrlBus
  TransitionDone : Inport  Port=2
  Action Port : ActionPort
  Bus Creator : BusCreator  Inputs=4  OutDataTypeStr=Bus: FixedWingCtrlBus
  Constant : Constant  Value=0
  Constant1 : Constant  Value=-0.2
  Constant2 : Constant  Value=0
  Constant3 : Constant  Value=0
  Switch : Switch  Criteria=u2 > Threshold  SaturateOnIntegerOverflow=off  InputSameDT=off
  FixedWingControls : Outport  OutDataTypeStr=Bus: FixedWingCtrlBus
  wires:
  Bus Creator/1 -> Switch/3
  Constant/1 -> Bus Creator/1  "dA"
  Constant1/1 -> Bus Creator/2  "dE"
  Constant2/1 -> Bus Creator/3  "dR"
  Constant3/1 -> Bus Creator/4  "dT"
  FixedWingActuators/1 -> Switch/1
  Switch/1 -> FixedWingControls/1
  TransitionDone/1 -> Switch/2

== system untitled1/Scheduler/FixedWingScheduler/Switch Case Action Subsystem2 ==
  FixedWingActuators : Inport  OutDataTypeStr=Bus: FixedWingCtrlBus
  Action Port : ActionPort
  FixedWingControls : Outport  OutDataTypeStr=Bus: FixedWingCtrlBus
  wires:
  FixedWingActuators/1 -> FixedWingControls/1

== system untitled1/Scheduler/FixedWingScheduler/Switch Case Action Subsystem3 ==
  note: No control allocated from fixed wing during hover.
  Action Port : ActionPort
  Bus Creator : BusCreator  Inputs=4
  Constant{,1..3} (4 alike) : Constant  Value=0
  FixedWingControls : Outport  OutDataTypeStr=Bus: FixedWingCtrlBus
  wires:
  Bus Creator/1 -> FixedWingControls/1
  Constant/1 -> Bus Creator/1  "dA"
  Constant1/1 -> Bus Creator/2  "dE"
  Constant3/1 -> Bus Creator/4  "dT"
  Constant2/1 -> Bus Creator/3  "dR"

== system untitled1/Scheduler/Subsystem/Actuator To Voltage ==
  Motor Commands : Inport
  Bus Creator : BusCreator  Inputs=6  OutDataTypeStr=Bus: RotorCtrlBus
  Bus Selector : BusSelector  OutputSignals=w1,w2,w3,w4,Tilt1,Tilt2
  Gain{,1..2,4} (4 alike) : Gain  Gain=1/(uavParam.motor.RPMMAX/60)
  Gain3 : Gain  Gain=1/(pi/2)
  Gain5 : Gain  Gain=1/(pi/2)
  To PWM : Outport
  wires:
  Motor Commands/1 -> Bus Selector/1
  Bus Selector/1 -> Gain/1  "<w1>"
  Bus Selector/3 -> Gain1/1  "<w3>"
  Bus Selector/2 -> Gain4/1  "<w2>"
  Bus Selector/4 -> Gain2/1  "<w4>"
  Bus Selector/5 -> Gain3/1  "<Tilt1>"
  Bus Selector/6 -> Gain5/1  "<Tilt2>"
  Gain/1 -> Bus Creator/1  "w1"
  Gain4/1 -> Bus Creator/2  "w2"
  Gain1/1 -> Bus Creator/3  "w3"
  Gain2/1 -> Bus Creator/4  "w4"
  Gain3/1 -> Bus Creator/5  "Tilt1"
  Gain5/1 -> Bus Creator/6  "Tilt2"
  Bus Creator/1 -> To PWM/1

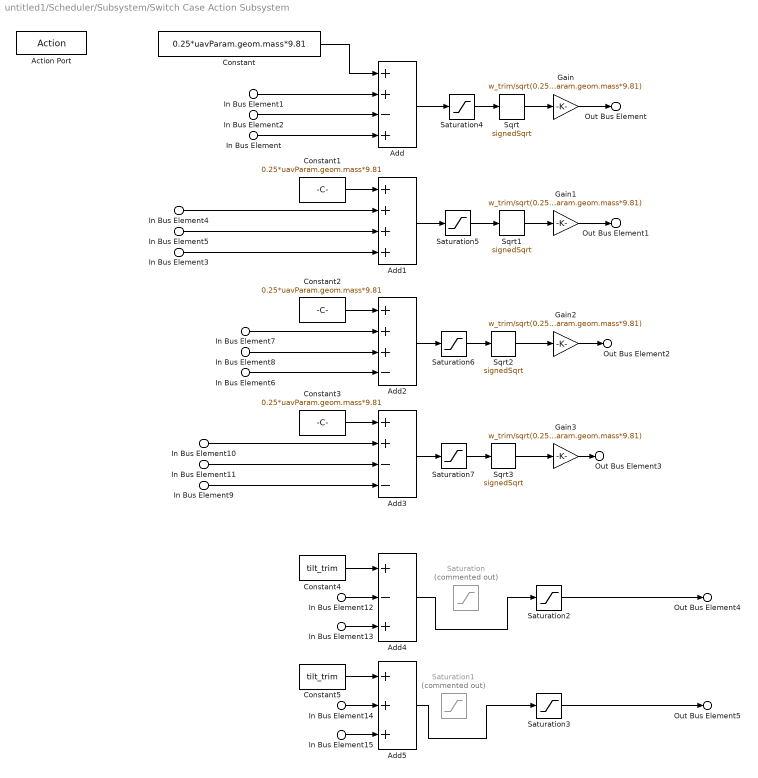
== system untitled1/Scheduler/Subsystem/Switch Case Action Subsystem ==
  In Bus Element{,3,6,9} (4 alike) : Inport  PortName=MixerCommands  Element=w_theta
  In Bus Element{1,4,7,10} (4 alike) : Inport  PortName=MixerCommands  Element=w_z
  In Bus Element{2,5,8,11} (4 alike) : Inport  PortName=MixerCommands  Element=w_phi
  In Bus Element12 : Inport  PortName=MixerCommands  Element=l_psi
  In Bus Element14 : Inport  PortName=MixerCommands  Element=l_psi
  In Bus Element13 : Inport  PortName=MixerCommands  Element=l_x
  In Bus Element15 : Inport  PortName=MixerCommands  Element=l_x
  Action Port : ActionPort
  Add : Sum  Inputs=++-+
  Add1 : Sum  Inputs=++++
  Add2 : Sum  Inputs=+++-
  Add3 : Sum  Inputs=++--
  Add4 : Sum  Inputs=+-+
  Add5 : Sum  Inputs=+++
  Constant{,1..3} (4 alike) : Constant  Value=0.25*uavParam.geom.mass*9.81
  Constant4 : Constant  Value=tilt_trim
  Constant5 : Constant  Value=tilt_trim
  Gain{,1..3} (4 alike) : Gain  Gain=w_trim/sqrt(0.25*uavParam.geom.mass*9.81)
  Saturation : Saturate  Commented=on  UpperLimit=tilt_max  LowerLimit=-tilt_max
  Saturation1 : Saturate  Commented=on  UpperLimit=tilt_max  LowerLimit=-tilt_max
  Saturation2 : Saturate  UpperLimit=tilt_max  LowerLimit=-tilt_max
  Saturation3 : Saturate  UpperLimit=tilt_max  LowerLimit=-tilt_max
  Saturation{4..7} (4 alike) : Saturate  UpperLimit=inf  LowerLimit=0
  Sqrt{,1..3} (4 alike) : Sqrt  Operator=signedSqrt
  Out Bus Element : Outport  PortName=Actuator  Element=w1
  Out Bus Element1 : Outport  PortName=Actuator  Element=w2
  Out Bus Element2 : Outport  PortName=Actuator  Element=w3
  Out Bus Element3 : Outport  PortName=Actuator  Element=w4
  Out Bus Element4 : Outport  PortName=Actuator  Element=Tilt1
  Out Bus Element5 : Outport  PortName=Actuator  Element=Tilt2
  wires:
  Constant5/1 -> Add5/1
  Constant2/1 -> Add2/1
  Constant1/1 -> Add1/1
  Constant4/1 -> Add4/1
  Constant/1 -> Add/1
  Constant3/1 -> Add3/1
  Add/1 -> Saturation4/1
  Add1/1 -> Saturation5/1
  Add2/1 -> Saturation6/1
  Add3/1 -> Saturation7/1
  In Bus Element12/1 -> Add4/2
  In Bus Element13/1 -> Add4/3
  In Bus Element14/1 -> Add5/2
  In Bus Element15/1 -> Add5/3
  Saturation2/1 -> Out Bus Element4/1
  Add4/1 -> Saturation2/1
  Add5/1 -> Saturation3/1
  Saturation3/1 -> Out Bus Element5/1
  Sqrt1/1 -> Gain1/1
  Sqrt2/1 -> Gain2/1
  Sqrt3/1 -> Gain3/1
  Saturation4/1 -> Sqrt/1
  Saturation5/1 -> Sqrt1/1
  Saturation6/1 -> Sqrt2/1
  Saturation7/1 -> Sqrt3/1
  Sqrt/1 -> Gain/1
  Gain/1 -> Out Bus Element/1
  Gain1/1 -> Out Bus Element1/1
  Gain2/1 -> Out Bus Element2/1
  Gain3/1 -> Out Bus Element3/1
  In Bus Element2/1 -> Add/3
  In Bus Element1/1 -> Add/2
  In Bus Element/1 -> Add/4
  In Bus Element4/1 -> Add1/2
  In Bus Element5/1 -> Add1/3
  In Bus Element3/1 -> Add1/4
  In Bus Element7/1 -> Add2/2
  In Bus Element8/1 -> Add2/3
  In Bus Element10/1 -> Add3/2
  In Bus Element11/1 -> Add3/3
  In Bus Element9/1 -> Add3/4
  In Bus Element6/1 -> Add2/4

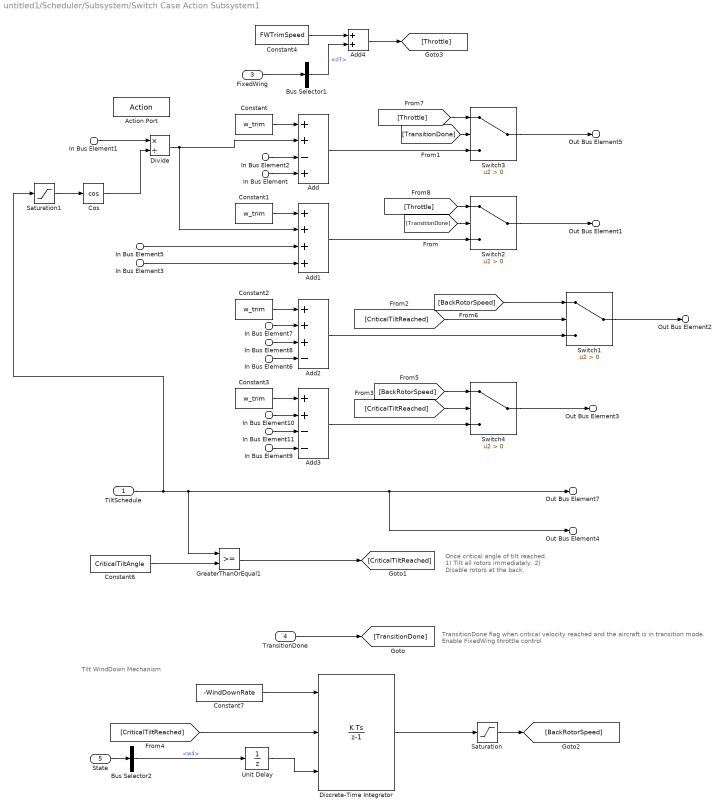
== system untitled1/Scheduler/Subsystem/Switch Case Action Subsystem1 ==
  note: Tilt WindDown Mechanism
  note: Once critical angle of tilt reached.
      | 1) Tilt all rotors immediately.
      | 2) Disable rotors at the back.
  note: TransitionDone flag when critical velocity reached and the aircraft is in transition mode.
      | Enable FixedWing throttle control
  TiltSchedule : Inport
  In Bus Element{,3,6,9} (4 alike) : Inport  Port=2  PortName=MixerCommands  Element=w_theta
  In Bus Element1 : Inport  Port=2  PortName=MixerCommands  Element=w_z
  In Bus Element7 : Inport  Port=2  PortName=MixerCommands  Element=w_z
  In Bus Element10 : Inport  Port=2  PortName=MixerCommands  Element=w_z
  In Bus Element{2,5,8,11} (4 alike) : Inport  Port=2  PortName=MixerCommands  Element=w_phi
  FixedWing : Inport  Port=3
  TransitionDone : Inport  Port=4
  State : Inport  Port=5
  Action Port : ActionPort
  Add : Sum  Inputs=++-+
  Add1 : Sum  Inputs=++++
  Add2 : Sum  Inputs=+++-
  Add3 : Sum  Inputs=++--
  Add4 : Sum
  Bus Selector1 : BusSelector  OutputSignals=dT
  Bus Selector2 : BusSelector  OutputSignals=RotorParameters.w4
  Constant{,1..3} (4 alike) : Constant  Value=w_trim
  Constant4 : Constant  Value=FWTrimSpeed
  Constant6 : Constant  Value=CriticalTiltAngle
  Constant7 : Constant  Value=-WindDownRate
  Cos : Trigonometry  Operator=cos
  Discrete-Time Integrator : DiscreteIntegrator  ExternalReset=either  InitialConditionSource=external  SampleTime=0.005  ICPrevOutput=DiscIntNeverNeededParam  ICPrevScaledInput=DiscIntNeverNeededParam
  Divide : Product  Inputs=*/
  GreaterThanOrEqual1 : RelationalOperator  OutDataTypeStr=boolean  RndMeth=Simplest  InputSameDT=off
  Saturation : Saturate  UpperLimit=Inf  LowerLimit=0
  Saturation1 : Saturate  UpperLimit=CriticalTiltAngle  LowerLimit=-CriticalTiltAngle
  Switch{1..4} (4 alike) : Switch  Criteria=u2 > Threshold  SaturateOnIntegerOverflow=off  InputSameDT=off
  Unit Delay : UnitDelay  SampleTime=-1  HasFrameUpgradeWarning=on
  Out Bus Element5 : Outport  PortName=Actuator  Element=w1
  Out Bus Element1 : Outport  PortName=Actuator  Element=w2
  Out Bus Element2 : Outport  PortName=Actuator  Element=w3
  Out Bus Element3 : Outport  PortName=Actuator  Element=w4
  Out Bus Element7 : Outport  PortName=Actuator  Element=Tilt1
  Out Bus Element4 : Outport  PortName=Actuator  Element=Tilt2
  wires:
  TiltSchedule/1 -> Saturation1/1, GreaterThanOrEqual1/1, Out Bus Element4/1, Out Bus Element7/1
  In Bus Element9/1 -> Add3/4
  In Bus Element6/1 -> Add2/4
  In Bus Element8/1 -> Add2/3
  Constant3/1 -> Add3/1
  In Bus Element/1 -> Add/4
  In Bus Element10/1 -> Add3/2
  Constant1/1 -> Add1/1
  In Bus Element11/1 -> Add3/3
  In Bus Element3/1 -> Add1/4
  In Bus Element2/1 -> Add/3
  In Bus Element7/1 -> Add2/2
  Constant2/1 -> Add2/1
  In Bus Element5/1 -> Add1/3
  Constant/1 -> Add/1
  [TransitionDone] -> Switch2/2
  FixedWing/1 -> Bus Selector1/1
  Bus Selector1/1 -> Add4/2  "<dT>"
  [TransitionDone] -> Switch3/2
  Constant6/1 -> GreaterThanOrEqual1/2
  GreaterThanOrEqual1/1 -> [CriticalTiltReached]
  [CriticalTiltReached] -> Switch1/2
  Add2/1 -> Switch1/3
  [BackRotorSpeed] -> Switch1/1
  [CriticalTiltReached] -> Switch4/2
  Add3/1 -> Switch4/3
  [BackRotorSpeed] -> Switch4/1
  TransitionDone/1 -> [TransitionDone]
  Bus Selector2/1 -> Unit Delay/1  "<w4>"
  Constant7/1 -> Discrete-Time Integrator/1
  [CriticalTiltReached] -> Discrete-Time Integrator/2
  Discrete-Time Integrator/1 -> Saturation/1
  Saturation/1 -> [BackRotorSpeed]
  State/1 -> Bus Selector2/1
  Unit Delay/1 -> Discrete-Time Integrator/3
  Constant4/1 -> Add4/1
  Add4/1 -> [Throttle]
  [Throttle] -> Switch3/1
  [Throttle] -> Switch2/1
  Add/1 -> Switch3/3
  Cos/1 -> Divide/2
  Add1/1 -> Switch2/3
  Saturation1/1 -> Cos/1
  In Bus Element1/1 -> Divide/1
  Divide/1 -> Add1/2, Add/2
  Switch3/1 -> Out Bus Element5/1
  Switch2/1 -> Out Bus Element1/1
  Switch1/1 -> Out Bus Element2/1
  Switch4/1 -> Out Bus Element3/1

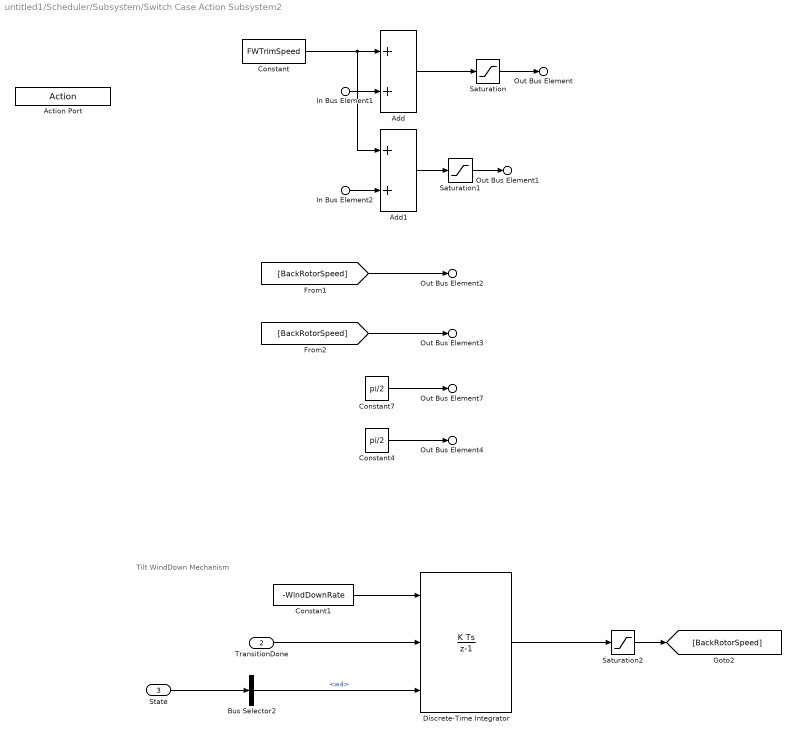
== system untitled1/Scheduler/Subsystem/Switch Case Action Subsystem2 ==
  note: Tilt WindDown Mechanism
  In Bus Element2 : Inport  PortName=FixedWingCtrlBus  Element=dT
  In Bus Element1 : Inport  PortName=FixedWingCtrlBus  Element=dT
  TransitionDone : Inport  Port=2
  State : Inport  Port=3
  Action Port : ActionPort
  Add : Sum
  Add1 : Sum
  Bus Selector2 : BusSelector  OutputSignals=RotorParameters.w4
  Constant : Constant  Value=FWTrimSpeed
  Constant1 : Constant  Value=-WindDownRate
  Constant4 : Constant  Value=pi/2
  Constant7 : Constant  Value=pi/2
  Discrete-Time Integrator : DiscreteIntegrator  ExternalReset=rising  InitialConditionSource=external  SampleTime=0.005  ICPrevOutput=DiscIntNeverNeededParam  ICPrevScaledInput=DiscIntNeverNeededParam
  Saturation : Saturate  UpperLimit=Inf  LowerLimit=0
  Saturation1 : Saturate  UpperLimit=Inf  LowerLimit=0
  Saturation2 : Saturate  UpperLimit=Inf  LowerLimit=0
  Out Bus Element : Outport  PortName=Actuator  Element=w1
  Out Bus Element1 : Outport  PortName=Actuator  Element=w2
  Out Bus Element2 : Outport  PortName=Actuator  Element=w3
  Out Bus Element3 : Outport  PortName=Actuator  Element=w4
  Out Bus Element7 : Outport  PortName=Actuator  Element=Tilt1
  Out Bus Element4 : Outport  PortName=Actuator  Element=Tilt2
  wires:
  Add1/1 -> Saturation1/1
  Constant4/1 -> Out Bus Element4/1
  [BackRotorSpeed] -> Out Bus Element2/1
  Constant/1 -> Add1/1, Add/1
  Constant7/1 -> Out Bus Element7/1
  In Bus Element2/1 -> Add1/2
  Add/1 -> Saturation/1
  In Bus Element1/1 -> Add/2
  Saturation/1 -> Out Bus Element/1
  Saturation1/1 -> Out Bus Element1/1
  [BackRotorSpeed] -> Out Bus Element3/1
  Bus Selector2/1 -> Discrete-Time Integrator/3  "<w4>"
  Saturation2/1 -> [BackRotorSpeed]
  State/1 -> Bus Selector2/1
  Constant1/1 -> Discrete-Time Integrator/1
  Discrete-Time Integrator/1 -> Saturation2/1
  TransitionDone/1 -> Discrete-Time Integrator/2

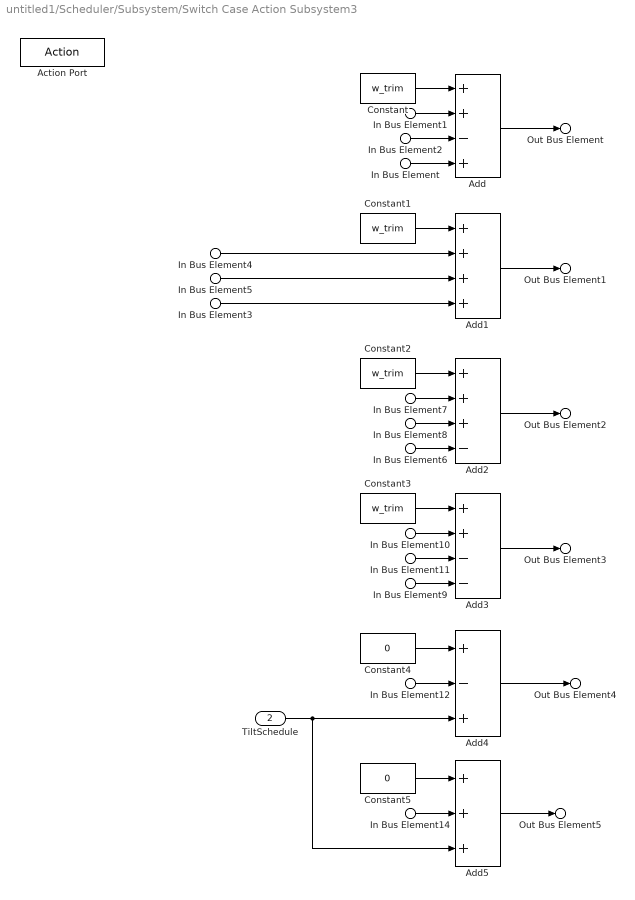
== system untitled1/Scheduler/Subsystem/Switch Case Action Subsystem3 ==
  In Bus Element{,3,6,9} (4 alike) : Inport  PortName=MixerCommands  Element=w_theta
  In Bus Element{1,4,7,10} (4 alike) : Inport  PortName=MixerCommands  Element=w_z
  In Bus Element{2,5,8,11} (4 alike) : Inport  PortName=MixerCommands  Element=w_phi
  In Bus Element12 : Inport  PortName=MixerCommands  Element=l_psi
  In Bus Element14 : Inport  PortName=MixerCommands  Element=l_psi
  TiltSchedule : Inport  Port=2
  Action Port : ActionPort
  Add : Sum  Inputs=++-+
  Add1 : Sum  Inputs=++++
  Add2 : Sum  Inputs=+++-
  Add3 : Sum  Inputs=++--
  Add4 : Sum  Inputs=+-+
  Add5 : Sum  Inputs=+++
  Constant{,1..3} (4 alike) : Constant  Value=w_trim
  Constant4 : Constant  Value=0
  Constant5 : Constant  Value=0
  Out Bus Element : Outport  PortName=Actuator  Element=w1
  Out Bus Element1 : Outport  PortName=Actuator  Element=w2
  Out Bus Element2 : Outport  PortName=Actuator  Element=w3
  Out Bus Element3 : Outport  PortName=Actuator  Element=w4
  Out Bus Element4 : Outport  PortName=Actuator  Element=Tilt1
  Out Bus Element5 : Outport  PortName=Actuator  Element=Tilt2
  wires:
  In Bus Element4/1 -> Add1/2
  In Bus Element2/1 -> Add/3
  In Bus Element5/1 -> Add1/3
  In Bus Element3/1 -> Add1/4
  In Bus Element/1 -> Add/4
  In Bus Element11/1 -> Add3/3
  In Bus Element8/1 -> Add2/3
  Constant2/1 -> Add2/1
  In Bus Element9/1 -> Add3/4
  In Bus Element6/1 -> Add2/4
  Constant1/1 -> Add1/1
  In Bus Element10/1 -> Add3/2
  In Bus Element1/1 -> Add/2
  Add1/1 -> Out Bus Element1/1
  Constant/1 -> Add/1
  Constant3/1 -> Add3/1
  Add/1 -> Out Bus Element/1
  Add2/1 -> Out Bus Element2/1
  Add3/1 -> Out Bus Element3/1
  In Bus Element7/1 -> Add2/2
  Constant4/1 -> Add4/1
  In Bus Element12/1 -> Add4/2
  TiltSchedule/1 -> Add5/3, Add4/3
  Constant5/1 -> Add5/1
  In Bus Element14/1 -> Add5/2
  Add4/1 -> Out Bus Element4/1
  Add5/1 -> Out Bus Element5/1

== system untitled1/Fixed Wing Controller/Fixed Wing Controller Module/Fixed Wing Controller Simulation/AER from Path Manager ==
  In1 : Inport
  Enable : EnablePort
  Out1 : Outport
  wires:
  In1/1 -> Out1/1
